simulink model "DR18E_Testpult"  (R2017a)
settings: Solver=ode1  StartTime=0.0  StopTime=Inf  FixedStep=0.001  RelTol=1e-3
PostLoadFcn:
  | , if any(exist('dsrtsu_mdlpostloadfcn', 'file') == [2, 3, 6]), try dsrtsu_mdlpostloadfcn('Execute', bdroot); catch fprintf('Error in PostLoadFcn (dsrtsu_mdlpostloadfcn) for model "%s":\n %s\n', bdroot, lasterr); end, end,
model workspace: external: MATLAB File C:\Users\DeltaRacing\Documents\dSPACE\MABX_DR18E\Model\DR18E_MABX_Parameter.m (data not in the file)
values from neighbouring files (symbols this model uses):
  am = 1/Ts    (= 1)    [DR18E_MABX_Parameter.m]
  bm = K/Ts    (= 0.05)    [DR18E_MABX_Parameter.m]
  cf = 41350    [DR18E_MABX_Parameter.m]
  cr = 41350    [DR18E_MABX_Parameter.m]
  Derating_HV_Battery_Kapa = 1    [DR18E_MABX_Parameter.m]
  Derating_Start_km = 16    [DR18E_MABX_Parameter.m]
  Drive_Mode = 0    [DR18E_MABX_Parameter.m]
  g = 1    [DR18E_MABX_Parameter.m]
  Gas_Modus = 2    [DR18E_MABX_Parameter.m]
  HV_Power_max = 80    [DR18E_MABX_Parameter.m]
  i_Getriebe = 3.3    [DR18E_MABX_Parameter.m]
  i_Lenkgetriebe = 4.32    [DR18E_MABX_Parameter.m]
  K_SET = 1    [DR18E_MABX_Parameter.m]
  Kapazitaet_HV_Battery_kWh = 6.6    [DR18E_MABX_Parameter.m]
  KW_T_Soll = 37    [DR18E_MABX_Parameter.m]
  lf = 1.2    [DR18E_MABX_Parameter.m]
  lr = 1.15    [DR18E_MABX_Parameter.m]
  m = 310    [DR18E_MABX_Parameter.m]
  M_max = 150    [DR18E_MABX_Parameter.m]
  Power_Limit_onoff = 0    [DR18E_MABX_Parameter.m]
  Reifenradius = 0.2351    [DR18E_MABX_Parameter.m]
  Strecke_Endu_km = 22    [DR18E_MABX_Parameter.m]
  TC_Decr_Gas = 0.00005    (= 5e-05)    [DR18E_MABX_Parameter.m]
  TC_Derivative = 0.4    [DR18E_MABX_Parameter.m]
  TC_Incr_Gas = 0.005    [DR18E_MABX_Parameter.m]
  TC_On = 0    [DR18E_MABX_Parameter.m]
  TC_Relay_Off = 0.065    [DR18E_MABX_Parameter.m]
  TC_Relay_On = 0.07    [DR18E_MABX_Parameter.m]
  TV_Mode = 2    [DR18E_MABX_Parameter.m]
  TV_On = 0    [DR18E_MABX_Parameter.m]
  TV_Override = 1    [DR18E_MABX_Parameter.m]
  y = 0.8    [DR18E_MABX_Parameter.m]
undefined symbols (not defined in the file or in its folder): D, DiscIntNeverNeededParam, I, K_OL, P
libraries: simulink x288, rtican x105, rtiusbflightreclib x40, rti1401lib_dio_type3 x10, simulink_extras x10, rti1401lib_adc_type4 x8, rti1401lib_II_base x7
(part 10 of 28)

== system DR18E_Testpult/Verarbeitung/BMS_Monitor ==
  In1 : Inport
  Bus Selector : BusSelector  OutputSignals=BMS,BMS_State,BMS.STK1-5_Temp
  Bus Selector1 : BusSelector  OutputSignals=Cell1-24.Cell1-12.Cell_Voltage_1,Cell1-24.Cell1-12.Cell_Voltage_2,Cell1-24.Cell1-12.Cell_Voltage_3,Cell1-24.Cell1-12.Cell_Voltage_4,Cell1-24.Cell1-12.Cell_Voltage_5,Cell1-24.Cell1-12.Cell_Voltage_6,Cell1-24.Cell1-12.Cell_Voltage_7,Cell1-24.Cell1-12.Cell_Voltage_8,Cell1-24.Cell1-12.Cell_Voltage_9,Cell1-24.Cell1-12.Cell_Voltage_10,Cell1-24.Cell1-12.Cell_Voltage_11,Cell1-24.Cell1-12.Cell_Voltage_12,HV_STR1_MIN_VOLTAGE,HV_STR1_MAX_VOLTAGE
  Bus Selector2 : BusSelector  OutputSignals=HV_Voltage_total,AMS_RelayState,AIR_minus_Status,AIR_plus_Status,Precharge_Relay_Status
  Bus Selector3 : BusSelector  OutputSignals=STK1_Temp1-5.STK1_Temp1,STK1_Temp1-5.STK1_Temp2,STK1_Temp1-5.STK1_Temp3,STK1_Temp1-5.STK1_Temp4,STK1_Temp1-5.STK1_Temp5
  Terminator{,1..23} (24 alike) : Terminator
  wires:
  In1/1 -> Bus Selector/1
  Bus Selector/1 -> Bus Selector1/1  "<BMS>"
  Bus Selector1/1 -> Terminator/1  "<Cell_Voltage_1>"
  Bus Selector1/2 -> Terminator1/1  "<Cell_Voltage_2>"
  Bus Selector1/3 -> Terminator2/1  "<Cell_Voltage_3>"
  Bus Selector1/4 -> Terminator3/1  "<Cell_Voltage_4>"
  Bus Selector1/5 -> Terminator4/1  "<Cell_Voltage_5>"
  Bus Selector1/6 -> Terminator6/1  "<Cell_Voltage_6>"
  Bus Selector1/7 -> Terminator5/1  "<Cell_Voltage_7>"
  Bus Selector1/8 -> Terminator7/1  "<Cell_Voltage_8>"
  Bus Selector1/9 -> Terminator8/1  "<Cell_Voltage_9>"
  Bus Selector1/10 -> Terminator9/1  "<Cell_Voltage_10>"
  Bus Selector1/11 -> Terminator10/1  "<Cell_Voltage_11>"
  Bus Selector1/12 -> Terminator13/1  "<Cell_Voltage_12>"
  Bus Selector1/13 -> Terminator12/1  "<HV_STR1_MIN_VOLTAGE>"
  Bus Selector1/14 -> Terminator11/1  "<HV_STR1_MAX_VOLTAGE>"
  Bus Selector/2 -> Bus Selector2/1  "<BMS_State>"
  Bus Selector2/1 -> Terminator14/1  "<HV_Voltage_total>"
  Bus Selector2/2 -> Terminator15/1  "<AMS_RelayState>"
  Bus Selector2/3 -> Terminator16/1  "<AIR_minus_Status>"
  Bus Selector2/4 -> Terminator17/1  "<AIR_plus_Status>"
  Bus Selector2/5 -> Terminator18/1  "<Precharge_Relay_Status>"
  Bus Selector/3 -> Bus Selector3/1  "<STK1-5_Temp>"
  Bus Selector3/4 -> Terminator22/1  "<STK1_Temp4>"
  Bus Selector3/1 -> Terminator19/1  "<STK1_Temp1>"
  Bus Selector3/2 -> Terminator20/1  "<STK1_Temp2>"
  Bus Selector3/3 -> Terminator21/1  "<STK1_Temp3>"
  Bus Selector3/5 -> Terminator23/1  "<STK1_Temp5>"

== system DR18E_Testpult/Verarbeitung/Bremse ==
  note: Wert: 0...250bar, 0.1 bar Auflösung
  note: 0x00: Alles Ok
      | 0xFF: Error, Sensoren Inplausibel
      | 0xEE: Error, zu hoher Messwert
      | 0xDD: Error, zu niedriger Messwert
      | 0xCC: Error, Kurzschluss
      | 0xBB: Error, Sensor fehlt
  Bremse : Inport
  Gaspedal % : Inport  Port=2
  Bus Selector : BusSelector  OutputSignals=Brake_vorne_1,Brake_rear_2
  Compare To Constant : simulink/Logic and Bit Operations/Compare To Constant  relop=>  const=3  OutDataTypeStr=boolean
  Constant1 : Constant
  FlightRecorder : Subsystem
  FlightRecorder1 : Subsystem
  FlightRecorder2 : Subsystem
  Logical Operator : Logic  Operator=OR  Inputs=1  AllPortsSameDT=off  OutDataTypeStr=boolean
  Mux1 : Mux  Inputs=2
  PT1 Discrete2 : Subsystem
  PlausibilityCheck : Subsystem
  TFilterGas1 : Constant  Value=0.1
  tag scope: Bremse_bin=global, W_Bemse_Inplausibel=global
  wires:
  Mux1/1 -> PT1 Discrete2/1(u)
  Gaspedal %/1 -> PlausibilityCheck/3(Gaspedal %)
  PT1 Discrete2/1(y) -> Compare To Constant/1
  TFilterGas1/1 -> PT1 Discrete2/3(T)
  Constant1/1 -> PT1 Discrete2/2(K)
  Bremse/1 -> Bus Selector/1
  Logical Operator/1 -> FlightRecorder2/1(In1), [Bremse_bin]  "Bremse_bin"
  Compare To Constant/1 -> Logical Operator/1
  Bus Selector/2 -> Mux1/2, PlausibilityCheck/2(Bremsdruck hinten), FlightRecorder1/1(In1)  "<Brake_rear_2>"
  Bus Selector/1 -> PlausibilityCheck/1(Bremsdruck vorne), Mux1/1, FlightRecorder/1(In1)  "<Brake_vorne_1>"
  PlausibilityCheck/1(W_Bremse_Inplausibel) -> [W_Bemse_Inplausibel]

== system DR18E_Testpult/Verarbeitung/DIS ==
  In1 : Inport
  Bus Creator : BusCreator  Inputs=1
  LED Bar Blinken Subsystem : Subsystem
  LED Bar Mode : Constant  OutDataTypeStr=boolean
  LED Bar blinken : Constant  OutDataTypeStr=boolean
  LED Farbe : Constant  Value=3
  Multiport Switch : MultiPortSwitch
  Mux : Mux  Inputs=8
  Out1 : Outport
  wires:
  LED Bar blinken/1 -> LED Bar Blinken Subsystem/1(LED Blinken)
  LED Farbe/1 -> LED Bar Blinken Subsystem/2(LED Farbe)
  LED Bar Blinken Subsystem/1(Out1) -> Mux/1, Mux/2, Mux/3, Mux/4, Mux/5, Mux/6, Mux/8, Mux/7
  Mux/1 -> Multiport Switch/2  "alle LED gleich"
  Bus Creator/1 -> Out1/1
  Multiport Switch/1 -> Bus Creator/1  "LED Bar Vektor"
  LED Bar Mode/1 -> Multiport Switch/1

== system DR18E_Testpult/Verarbeitung/DR18E Torque Control ==
  Gas_0-1 : Inport
  Inputs : Inport  Port=2
  Add : Sum
  Add1 : Sum
  Bus Creator : BusCreator  Inputs=7
  Derating : Subsystem
  FlightRecorder : Subsystem
  Gain2 : Gain  Gain=-g
  Gain4 : Gain  Gain=g
  M Max : Constant  Value=M_max
  M_max : Constant  Value=M_max
  Mux : Mux  Inputs=2
  Power Limit : Subsystem
  Power Limit onoff : Constant  Value=Power_Limit_onoff
  Product : Product
  Product1 : Product
  Saturation : Saturate  UpperLimit=0  LowerLimit=-M_max
  Saturation1 : Saturate  UpperLimit=M_max  LowerLimit=0
  Saturation2 : Saturate  UpperLimit=0  LowerLimit=-M_max
  Saturation3 : Saturate  UpperLimit=M_max  LowerLimit=0
  TC RL : Subsystem
  TC RR : Subsystem
  TC on : Constant  Value=TC_On
  TV RL : Subsystem
  TV RR : Subsystem
  Torque Filter : Subsystem
  MotorTorque Nm : Outport
  M_max/Motor : Outport  Port=2
  Logs2 : Outport  Port=3
  wires:
  Add/1 -> Saturation1/1
  Gain2/1 -> Saturation/1  "Torque_RL-"
  TC RL/2(Motor_Gas_RL) -> Product/2
  Product/1 -> Add/1
  TV RL/1(TV RL Nm) -> Gain2/1
  Saturation/1 -> Add/2
  Gas_0-1/1 -> TC RR/2(Gas_0-1), TC RL/2(Gas_0-1)
  Saturation1/1 -> Power Limit/2(DriverTorqueRequest L [Nm])  "TQ_left_after_TCTV_Nm"
  Saturation3/1 -> Power Limit/3(DriverTorqueRequest R [Nm])  "TQ_right_after_TCTV_Nm"
  Inputs/1 -> Power Limit/4(Inputs), Derating/1(In1), TV RR/1(Inputs), TC RR/3(Inputs), TV RL/1(Inputs), TC RL/3(Inputs)
  Bus Creator/1 -> Logs2/1
  Add1/1 -> Saturation3/1
  TC RR/2(Motor_Gas_RR) -> Product1/2
  Saturation2/1 -> Add1/2
  Product1/1 -> Add1/1
  TC on/1 -> TC RR/1(TC_On), TC RL/1(TC_On)
  TV RR/1(TV RR Nm) -> Gain4/1
  Gain4/1 -> Saturation2/1
  Power Limit/2(LimitedTorque R [Nm]) -> Mux/2
  Power Limit/1(LimitedTorque L [Nm]) -> Mux/1
  Mux/1 -> MotorTorque Nm/1  "Torque_after_PowerLimit_Nm"
  M_max/1 -> Bus Creator/1
  M Max/1 -> FlightRecorder/1(In1), M_max/Motor/1, Product1/1, Product/1  "MmaxproMotor"
  Derating/1(PowerLimit_kW) -> Power Limit/5(Power Limit kW)
  Power Limit onoff/1 -> Power Limit/1(Power Limit onoff)

== system DR18E_Testpult/Verarbeitung/GLV-Undervoltage ==
  GLV-Spannung : Inport
  Bus Selector12 : BusSelector  OutputSignals=RX_GLVAMS.GLV_Voltage_ges
  Cubatt : Constant  Value=0
  Pulse Generator : DiscretePulseGenerator  PulseType=Time based  Period=1  PulseWidth=20
  Switch : Switch  Threshold=11
  GLV-Undervoltage : Outport
  wires:
  Pulse Generator/1 -> Switch/3
  Switch/1 -> GLV-Undervoltage/1  "LV_Undervoltage"
  Cubatt/1 -> Switch/1
  GLV-Spannung/1 -> Bus Selector12/1
  Bus Selector12/1 -> Switch/2  "<GLV_Voltage_ges>"

== system DR18E_Testpult/Verarbeitung/Gaspedal Check ==
  note: 0x00: Alles Ok
      | 0xFF: Error, Sensoren Inplausibel
      | 0xEE: Error, zu hoher Messwert
      | 0xDD: Error, zu niedriger Messwert
      | 0xCC: Error, Kurzschluss
      | 0xBB: Error, Sensor fehlt
      | 0xAA: Sensoren Inplausibel (Erkennung in Software)
  note: 0...100.0% (0.1% Auflösung)
  Gaspedal : Inport
  Add_Software_inplausible_Warning : Subsystem
  Add_Software_inplausible_Warning1 : Subsystem
  Bus Selector : BusSelector  OutputSignals=RX_SensorboardFront.RX_Gas.Throttle_1,RX_SensorboardFront.RX_Gas.Throttle_2,RX_SensorboardFront.RX_Gas.Throttle_1_Status,RX_SensorboardFront.RX_Gas.Throttle_2_Status,RX_SensorboardFront.RX_Gas.RX Timeout Error
  FlightRecorder : Subsystem
  Gas_Modus : Constant  Value=Gas_Modus
  Multiport Switch : MultiPortSwitch  Inputs=2
  PlausibilityCheck : Subsystem
  Saturation 0-1 : Saturate  UpperLimit=1  LowerLimit=0
  Testmodus : Subsystem
  Gas_0-1 : Outport
  tag scope: A_Gas_RX_Timeout=global, W_Gas1_Error=global, W_Gas2_Error=global
  wires:
  Bus Selector/1 -> Testmodus/1(Gas1), PlausibilityCheck/1(Gas1)  "<Throttle_1>"
  Bus Selector/2 -> Testmodus/2(Gas2), PlausibilityCheck/2(Gas2)  "<Throttle_2>"
  Add_Software_inplausible_Warning/1(ErrorCode_Out) -> [W_Gas1_Error]
  Bus Selector/3 -> Add_Software_inplausible_Warning/2(Error_Code)  "<Throttle_1_Status>"
  Add_Software_inplausible_Warning1/1(ErrorCode_Out) -> [W_Gas2_Error]
  Bus Selector/4 -> Add_Software_inplausible_Warning1/2(Error_Code)  "<Throttle_2_Status>"
  Bus Selector/5 -> [A_Gas_RX_Timeout]  "<RX Timeout Error>"
  Gaspedal/1 -> Bus Selector/1
  Saturation 0-1/1 -> Gas_0-1/1, Add_Software_inplausible_Warning1/1(Softw_Plausibel), Add_Software_inplausible_Warning/1(Softw_Plausibel)  "Gas_0-1"
  Multiport Switch/1 -> FlightRecorder/1(In1), Saturation 0-1/1
  Gas_Modus/1 -> Multiport Switch/1
  PlausibilityCheck/1(Gas_0-1_plausibel) -> Multiport Switch/3
  Testmodus/1(Gas_0-1) -> Multiport Switch/2

== system DR18E_Testpult/Verarbeitung/MABX RAM ==
  In1 : Inport
  Add : Sum
  Add1 : Sum
  Add2 : Sum
  Data Type Conversion : DataTypeConversion  OutDataTypeStr=uint16
  Data Type Conversion1 : DataTypeConversion  OutDataTypeStr=uint32
  Data Type Conversion2 : DataTypeConversion  OutDataTypeStr=uint16
  Difference : simulink/Discrete/Difference  ICPrevInput=0.0  OutMin=[]  OutMax=[]  OutDataType=fixdt(1, 16)  OutScaling=2^-10  DoSatur=off
  Difference1 : simulink/Discrete/Difference  ICPrevInput=0.0  OutMin=[]  OutMax=[]  OutDataType=fixdt(1, 16)  OutScaling=2^-10  DoSatur=off
  Difference2 : simulink/Discrete/Difference  ICPrevInput=0.0  OutMin=[]  OutMax=[]  OutDataType=fixdt(1, 16)  OutScaling=2^-10  DoSatur=off
  FlightRecorder5 : Subsystem
  READ Gesamtkilometerzähler Byte 1+2 : rti1401lib_II_base/DS1401_NV_RAM_READ_BL1  DSProperties=struct('RTI',struct('Version',uint32(1),'BlockType',struct('isSLSource',uint8(1),'isSLSink',uint8(0),'isHWSource',uint8(1),'isHWSink',uint8(0),'isSetup',uint8(0),'isInline',uint8(1),'isNonInline',uint8(0),'isInterrupt',uint8(0),'isChannelwise',uint8(0)),'IOBoardType',{{'DS1401','BASE','II'}},'UnitType','NVRAM','Identifier','NVRAMREAD','DialogType','ML','BlockSet','NONE','SlaveProcessor','NONE'))  RTIBlockInterface=struct('OutputPortsWidth',int32(1),'OutputPortsActive',1,'OutputPortsDataType',{{'SS_UINT16'}},'OutputPortsName',{{[' ']}},'BlockDisplay',{{['Read from\nnon-volatile RAM'],'center'}},'IconTransparency','on','InitLevel',3,'SampleTime',{{-1}},'DialogFcn','rti1401baseiinvramreadgui','BlockName',struct('Token',{{'DS1401_NV_RAM_READ_BL1'}}))  RTIBlockParameters=struct('DataType',{{4,'OFF',[1 8]}},'RAMAddress',{{'1','OFF',[0 4095]}},'SampleTime',{{'-1','OFF',[-1 inf]}},'TLCFileName',{{'rti1401base_II_nvram_read','OFF',[]}})  RTISFcnParameters=struct('DataType','int16','RAMAddress','uint32','TLCFileName','char')  RTIBlockParaDefault=struct('DataType',8,'RAMAddress',0,'SampleTime',-1,'TLCFileName','rti1401base_II_nvram_read')
  READ Gesamtkilometerzähler Byte 10+4 : rti1401lib_II_base/DS1401_NV_RAM_READ_BL1  DSProperties=struct('RTI',struct('Version',uint32(1),'BlockType',struct('isSLSource',uint8(1),'isSLSink',uint8(0),'isHWSource',uint8(1),'isHWSink',uint8(0),'isSetup',uint8(0),'isInline',uint8(1),'isNonInline',uint8(0),'isInterrupt',uint8(0),'isChannelwise',uint8(0)),'IOBoardType',{{'DS1401','BASE','II'}},'UnitType','NVRAM','Identifier','NVRAMREAD','DialogType','ML','BlockSet','NONE','SlaveProcessor','NONE'))  RTIBlockInterface=struct('OutputPortsWidth',int32(1),'OutputPortsActive',1,'OutputPortsDataType',{{'SS_UINT32'}},'OutputPortsName',{{[' ']}},'BlockDisplay',{{['Read from\nnon-volatile RAM'],'center'}},'IconTransparency','on','InitLevel',3,'SampleTime',{{-1}},'DialogFcn','rti1401baseiinvramreadgui','BlockName',struct('Token',{{'DS1401_NV_RAM_READ_BL1'}}))  RTIBlockParameters=struct('DataType',{{6,'OFF',[1 8]}},'RAMAddress',{{'10','OFF',[0 4095]}},'SampleTime',{{'-1','OFF',[-1 inf]}},'TLCFileName',{{'rti1401base_II_nvram_read','OFF',[]}})  RTISFcnParameters=struct('DataType','int16','RAMAddress','uint32','TLCFileName','char')  RTIBlockParaDefault=struct('DataType',8,'RAMAddress',0,'SampleTime',-1,'TLCFileName','rti1401base_II_nvram_read')
  READ Tagesenergiezähler Byte 4+2 : rti1401lib_II_base/DS1401_NV_RAM_READ_BL1  DSProperties=struct('RTI',struct('Version',uint32(1),'BlockType',struct('isSLSource',uint8(1),'isSLSink',uint8(0),'isHWSource',uint8(1),'isHWSink',uint8(0),'isSetup',uint8(0),'isInline',uint8(1),'isNonInline',uint8(0),'isInterrupt',uint8(0),'isChannelwise',uint8(0)),'IOBoardType',{{'DS1401','BASE','II'}},'UnitType','NVRAM','Identifier','NVRAMREAD','DialogType','ML','BlockSet','NONE','SlaveProcessor','NONE'))  RTIBlockInterface=struct('OutputPortsWidth',int32(1),'OutputPortsActive',1,'OutputPortsDataType',{{'SS_UINT16'}},'OutputPortsName',{{[' ']}},'BlockDisplay',{{['Read from\nnon-volatile RAM'],'center'}},'IconTransparency','on','InitLevel',3,'SampleTime',{{-1}},'DialogFcn','rti1401baseiinvramreadgui','BlockName',struct('Token',{{'DS1401_NV_RAM_READ_BL1'}}))  RTIBlockParameters=struct('DataType',{{4,'OFF',[1 8]}},'RAMAddress',{{'4','OFF',[0 4095]}},'SampleTime',{{'-1','OFF',[-1 inf]}},'TLCFileName',{{'rti1401base_II_nvram_read','OFF',[]}})  RTISFcnParameters=struct('DataType','int16','RAMAddress','uint32','TLCFileName','char')  RTIBlockParaDefault=struct('DataType',8,'RAMAddress',0,'SampleTime',-1,'TLCFileName','rti1401base_II_nvram_read')
  Reset Tageswerte : Constant  Value=0
  Reset Value : Constant  Value=0  OutDataTypeStr=uint16
  Reset Value1 : Constant  Value=0  OutDataTypeStr=uint16
  Switch : Switch  Criteria=u2 > Threshold
  Switch1 : Switch  Criteria=u2 > Threshold
  WRITE Gesamtmeterzähler m Byte 10+4 : rti1401lib_II_base/DS1401_NV_RAM_WRITE_BL1  DSProperties=struct('RTI',struct('Version',uint32(1),'BlockType',struct('isSLSource',uint8(0),'isSLSink',uint8(1),'isHWSource',uint8(0),'isHWSink',uint8(1),'isSetup',uint8(0),'isInline',uint8(1),'isNonInline',uint8(0),'isInterrupt',uint8(0),'isChannelwise',uint8(0)),'IOBoardType',{{'DS1401','BASE','II'}},'UnitType','NVRAM','Identifier','NVRAMWRITE','DialogType','ML','BlockSet','NONE','SlaveProcessor','NONE'))  RTIBlockInterface=struct('InputPortsWidth',int32(1),'InputPortsActive',1,'InputPortsDataType',{{'SS_UINT32'}},'InputPortsName',{{[' ']}},'BlockDisplay',{{['Write to\nnon-volatile RAM'],'center'}},'IconTransparency','on','InitLevel',3,'SampleTime',{{-1}},'DialogFcn','rti1401baseiinvramwritegui','BlockName',struct('Token',{{'DS1401_NV_RAM_WRITE_BL1'}}))  RTIBlockParameters=struct('DataType',{{6,'OFF',[1 8]}},'RAMAddress',{{'10','OFF',[0 4095]}},'SampleTime',{{'-1','OFF',[-1 inf]}},'TLCFileName',{{'rti1401base_II_nvram_write','OFF',[]}})  RTISFcnParameters=struct('DataType','int16','RAMAddress','uint32','TLCFileName','char')  RTIBlockParaDefault=struct('DataType',8,'RAMAddress',0,'SampleTime',-1,'TLCFileName','rti1401base_II_nvram_write')
  WRITE Tagesmeterzähler Wh Byte 4+2 : rti1401lib_II_base/DS1401_NV_RAM_WRITE_BL1  DSProperties=struct('RTI',struct('Version',uint32(1),'BlockType',struct('isSLSource',uint8(0),'isSLSink',uint8(1),'isHWSource',uint8(0),'isHWSink',uint8(1),'isSetup',uint8(0),'isInline',uint8(1),'isNonInline',uint8(0),'isInterrupt',uint8(0),'isChannelwise',uint8(0)),'IOBoardType',{{'DS1401','BASE','II'}},'UnitType','NVRAM','Identifier','NVRAMWRITE','DialogType','ML','BlockSet','NONE','SlaveProcessor','NONE'))  RTIBlockInterface=struct('InputPortsWidth',int32(1),'InputPortsActive',1,'InputPortsDataType',{{'SS_UINT16'}},'InputPortsName',{{[' ']}},'BlockDisplay',{{['Write to\nnon-volatile RAM'],'center'}},'IconTransparency','on','InitLevel',3,'SampleTime',{{-1}},'DialogFcn','rti1401baseiinvramwritegui','BlockName',struct('Token',{{'DS1401_NV_RAM_WRITE_BL1'}}))  RTIBlockParameters=struct('DataType',{{4,'OFF',[1 8]}},'RAMAddress',{{'4','OFF',[0 4095]}},'SampleTime',{{'-1','OFF',[-1 inf]}},'TLCFileName',{{'rti1401base_II_nvram_write','OFF',[]}})  RTISFcnParameters=struct('DataType','int16','RAMAddress','uint32','TLCFileName','char')  RTIBlockParaDefault=struct('DataType',8,'RAMAddress',0,'SampleTime',-1,'TLCFileName','rti1401base_II_nvram_write')
  WRITE Tagesmeterzähler m Byte 1+2 : rti1401lib_II_base/DS1401_NV_RAM_WRITE_BL1  DSProperties=struct('RTI',struct('Version',uint32(1),'BlockType',struct('isSLSource',uint8(0),'isSLSink',uint8(1),'isHWSource',uint8(0),'isHWSink',uint8(1),'isSetup',uint8(0),'isInline',uint8(1),'isNonInline',uint8(0),'isInterrupt',uint8(0),'isChannelwise',uint8(0)),'IOBoardType',{{'DS1401','BASE','II'}},'UnitType','NVRAM','Identifier','NVRAMWRITE','DialogType','ML','BlockSet','NONE','SlaveProcessor','NONE'))  RTIBlockInterface=struct('InputPortsWidth',int32(1),'InputPortsActive',1,'InputPortsDataType',{{'SS_UINT16'}},'InputPortsName',{{[' ']}},'BlockDisplay',{{['Write to\nnon-volatile RAM'],'center'}},'IconTransparency','on','InitLevel',3,'SampleTime',{{-1}},'DialogFcn','rti1401baseiinvramwritegui','BlockName',struct('Token',{{'DS1401_NV_RAM_WRITE_BL1'}}))  RTIBlockParameters=struct('DataType',{{4,'OFF',[1 8]}},'RAMAddress',{{'1','OFF',[0 4095]}},'SampleTime',{{'-1','OFF',[-1 inf]}},'TLCFileName',{{'rti1401base_II_nvram_write','OFF',[]}})  RTISFcnParameters=struct('DataType','int16','RAMAddress','uint32','TLCFileName','char')  RTIBlockParaDefault=struct('DataType',8,'RAMAddress',0,'SampleTime',-1,'TLCFileName','rti1401base_II_nvram_write')
  TagesmeterMABX_m : Outport
  TagesenergieMABX_Wh : Outport  Port=2
  wires:
  READ Gesamtkilometerzähler Byte 10+4/1 -> Add/2
  Add/1 -> FlightRecorder5/1(In1), WRITE Gesamtmeterzähler m Byte 10+4/1
  [Tagesmeter_s_m] -> Data Type Conversion1/1
  Difference/1 -> Add/1
  Difference1/1 -> Add1/1
  READ Gesamtkilometerzähler Byte 1+2/1 -> Add1/2
  [Tagesmeter_s_m] -> Data Type Conversion/1
  Add1/1 -> Switch/3
  Switch/1 -> TagesmeterMABX_m/1, WRITE Tagesmeterzähler m Byte 1+2/1  "TagesmeterMABX_m"
  Reset Tageswerte/1 -> Switch/2, Switch1/2  "Reset Tageswerte"
  Reset Value/1 -> Switch/1
  Data Type Conversion/1 -> Difference1/1
  Data Type Conversion1/1 -> Difference/1
  READ Tagesenergiezähler Byte 4+2/1 -> Add2/2
  Difference2/1 -> Add2/1
  Switch1/1 -> TagesenergieMABX_Wh/1, WRITE Tagesmeterzähler Wh Byte 4+2/1  "TagesenergieMABX_Wh"
  Add2/1 -> Switch1/3
  Reset Value1/1 -> Switch1/1
  [Tages_HV_energy_con_Wh] -> Data Type Conversion2/1
  Data Type Conversion2/1 -> Difference2/1

== system DR18E_Testpult/Verarbeitung/Precalculations ==
  Drehzahl FL : Inport
  Drehzahl FR : Inport  Port=2
  Drehzahl RL : Inport  Port=3
  Drehzahl RR : Inport  Port=4
  "Inputs Bus " : Inport  Port=5
  Bus Creator : BusCreator  Inputs=3
  FlightRecorder : Subsystem
  FlightRecorder1 : Subsystem
  FlightRecorder2 : Subsystem
  FlightRecorder3 : Subsystem
  FlightRecorder4 : Subsystem
  FlightRecorder5 : Subsystem
  FlightRecorder6 : Subsystem
  Gain : Gain  Gain=1/i_Getriebe
  Gain1 : Gain  Gain=1/i_Getriebe
  Mux : Mux  Inputs=2
  Mux1 : Mux  Inputs=2
  Saturation : Saturate  UpperLimit=1  LowerLimit=0
  Saturation1 : Saturate  UpperLimit=1  LowerLimit=0
  Sum : Sum  Inputs=|++
  Wheelslip Calculation Left : Fcn  Expr=-(u(1) - u(2))/(abs(u(2)) + 0.1)
  Wheelslip Calulation Right : Fcn  Expr=-(u(1) - u(2))/(abs(u(2)) + 0.1)
  größer 0 : Saturate  UpperLimit=100  LowerLimit=0
  kilometer tracking : Subsystem
  "m/s -> km/h" : Gain  Gain=3.6
  rpm-rad/s : Gain  Gain=2*pi/60
  rpm-rad/s1 : Gain  Gain=2*pi/60
  v = omega*r : Gain  Gain=0.5 * 2* pi *(1/60)*Reifenradius
  v_kmh : Outport
  Long_Slip_Left : Outport  Port=2
  Long_Slip_Right : Outport  Port=3
  Outputs Bus : Outport  Port=4
  wires:
  Drehzahl FL/1 -> FlightRecorder4/1(In1), Mux/1, Sum/1  "Drehzahl_FL_rpm"
  Drehzahl FR/1 -> FlightRecorder3/1(In1), Mux1/1, Sum/2  "Drehzahl_FR_rpm"
  Sum/1 -> v = omega*r/1
  v = omega*r/1 -> größer 0/1, "m/s -> km/h"/1
  Mux/1 -> Wheelslip Calculation Left/1
  Drehzahl RL/1 -> rpm-rad/s/1, Gain/1  "Drehzahl_RL_rpm"
  Wheelslip Calculation Left/1 -> Saturation/1
  Mux1/1 -> Wheelslip Calulation Right/1
  Wheelslip Calulation Right/1 -> Saturation1/1
  Drehzahl RR/1 -> rpm-rad/s1/1, Gain1/1  "Drehzahl_RR_rpm"
  Gain/1 -> Mux/2, FlightRecorder1/1(In1)
  Gain1/1 -> Mux1/2, FlightRecorder2/1(In1)
  Saturation/1 -> FlightRecorder5/1(In1), Long_Slip_Left/1
  Saturation1/1 -> Long_Slip_Right/1, FlightRecorder6/1(In1)
  "m/s -> km/h"/1 -> FlightRecorder/1(In1), v_kmh/1
  Bus Creator/1 -> Outputs Bus/1
  "Inputs Bus "/1 -> Bus Creator/3
  rpm-rad/s/1 -> Bus Creator/1  "Drehzahl_RL_rad/s"
  rpm-rad/s1/1 -> Bus Creator/2  "Drehzahl_RR_rad/s"
  größer 0/1 -> kilometer tracking/1(v_ms)

== system DR18E_Testpult/Verarbeitung/SafetyShutdown ==
  TorqueRequestLR : Inport
  Constant : Constant  Value=[0;0]
  Constant1 : Constant  Value=0
  Gas_Modus : Constant  Value=Gas_Modus
  Multiport Switch : MultiPortSwitch  Inputs=2
  Switch : Switch  Criteria=u2 > Threshold
  TorqueRequestLROut : Outport
  wires:
  TorqueRequestLR/1 -> Switch/3
  Constant/1 -> Switch/1
  Switch/1 -> TorqueRequestLROut/1
  Gas_Modus/1 -> Multiport Switch/1
  Constant1/1 -> Multiport Switch/2
  Multiport Switch/1 -> Switch/2
  [Warnings] -> Multiport Switch/3

== system DR18E_Testpult/Verarbeitung/Strom//SOC ==
  HV_Voltage : Inport
  HV_Current : Inport  Port=2
  Discrete-Time Integrator : DiscreteIntegrator  ICPrevOutput=DiscIntNeverNeededParam  ICPrevScaledInput=DiscIntNeverNeededParam
  Discrete-Time Integrator1 : DiscreteIntegrator  ICPrevOutput=DiscIntNeverNeededParam  ICPrevScaledInput=DiscIntNeverNeededParam
  HVIRecorder : Subsystem
  HVURecorder : Subsystem
  Product : Product
  Ws->Wh : Gain  Gain=1/3600
  currentConsumptionRecorder : Subsystem
  powerConsumtionRecorder : Subsystem
  powerRecorder : Subsystem
  HV_Power_Watt : Outport
  tag scope: Tages_HV_energy_con_Wh=global
  wires:
  HV_Voltage/1 -> Product/1, HVURecorder/1(In1)  "HV_Voltage"
  HV_Current/1 -> Discrete-Time Integrator/1, Product/2, HVIRecorder/1(In1)  "HV_Current"
  Discrete-Time Integrator/1 -> currentConsumptionRecorder/1(In1)  "CurrentConsumption"
  Product/1 -> Discrete-Time Integrator1/1, HV_Power_Watt/1, powerRecorder/1(In1)  "HV_Power_Watt"
  Discrete-Time Integrator1/1 -> Ws->Wh/1, powerConsumtionRecorder/1(In1)  "HV_energy_con_Ws"
  Ws->Wh/1 -> [Tages_HV_energy_con_Wh]

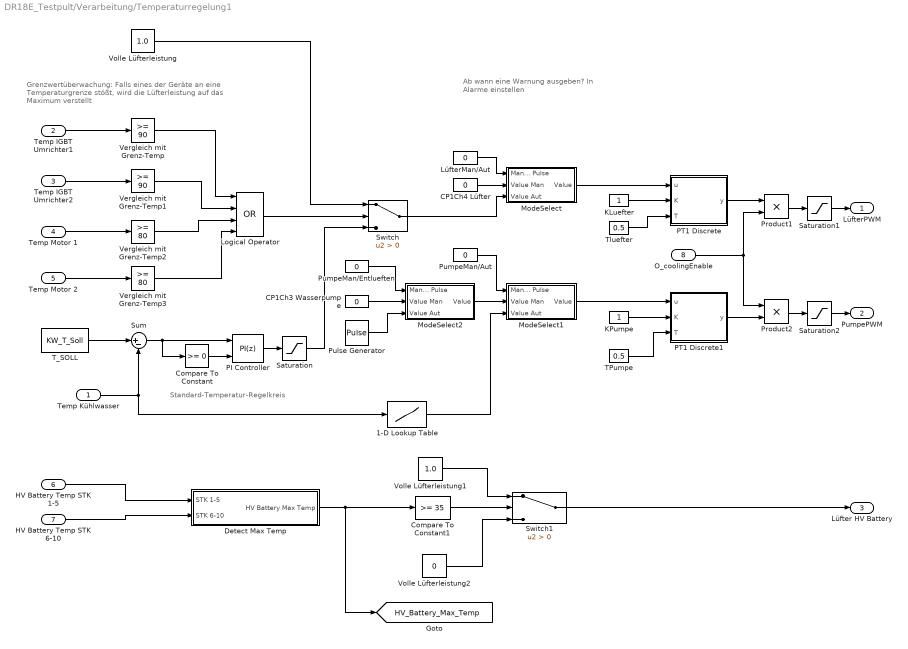
== system DR18E_Testpult/Verarbeitung/Temperaturregelung1 ==
  note: Ab wann eine Warnung ausgeben?
      |
      | In Alarme einstellen
  note: Grenzwertüberwachung:
      | Falls eines der Geräte an eine Temperaturgrenze stößt,
      | wird die Lüfterleistung auf das Maximum verstellt
  note: Standard-Temperatur-Regelkreis
  Temp Kühlwasser : Inport
  Temp IGBT Umrichter1 : Inport  Port=2
  Temp IGBT Umrichter2 : Inport  Port=3
  Temp Motor 1 : Inport  Port=4
  Temp Motor 2 : Inport  Port=5
  HV Battery Temp STK 1-5 : Inport  Port=6
  HV Battery Temp STK 6-10 : Inport  Port=7
  O_coolingEnable : Inport  Port=8
  1-D Lookup Table : Lookup_n-D  NumberOfTableDimensions=1  BreakpointsForDimension1=[0,20,28,35,40,45,50,100]  Table=[0.2,0.2,0.2,0.4,0.6,0.8,1,1]  RndMeth=Simplest  InputSameDT=on
  CP1Ch3 Wasserpumpe : Constant  Value=0
  CP1Ch4 Lüfter : Constant  Value=0
  Compare To Constant : simulink/Logic and Bit Operations/Compare To Constant  relop=>=  const=0  OutDataTypeStr=boolean
  Compare To Constant1 : simulink/Logic and Bit Operations/Compare To Constant  relop=>=  const=35  OutDataTypeStr=boolean
  Detect Max Temp : Subsystem
  KLuefter : Constant
  KPumpe : Constant
  Logical Operator : Logic  Operator=OR  Inputs=4  AllPortsSameDT=off  OutDataTypeStr=boolean
  LüfterMan/Aut : Constant  Value=0
  ModeSelect : Subsystem
  ModeSelect1 : Subsystem
  ModeSelect2 : Subsystem
  PI Controller : simulink/Continuous/PID Controller  Controller=PI  TimeDomain=Discrete-time  SampleTime=0.2  IntegratorMethod=Forward Euler  FilterMethod=Forward Euler  Form=Parallel  UseFilter=on  ControllerParametersSource=internal  P=-0.02  I=-0.01  D=0  N=100  InitialConditionSource=internal  InitialConditionForIntegrator=0  InitialConditionForFilter=0  ExternalReset=level  LimitOutput=off  UpperSaturationLimit=inf  LowerSaturationLimit=-inf  LinearizeAsGain=on  AntiWindupMode=none  Kb=1  TrackingMode=off  Kt=1  PParamMin=[]  PParamMax=[]  IParamMin=[]  IParamMax=[]  DParamMin=[]  DParamMax=[]  NParamMin=[]  NParamMax=[]  KbParamMin=[]  KbParamMax=[]  KtParamMin=[]  KtParamMax=[]  POutMin=[]  POutMax=[]  IOutMin=[]  IOutMax=[]  DOutMin=[]  DOutMax=[]  NOutMin=[]  NOutMax=[]  KbOutMin=[]  KbOutMax=[]  KtOutMin=[]  KtOutMax=[]  IntegratorOutMin=[]  IntegratorOutMax=[]  FilterOutMin=[]  FilterOutMax=[]  SumOutMin=[]  SumOutMax=[]  SumI1OutMin=[]  SumI1OutMax=[]  SumI2OutMin=[]  SumI2OutMax=[]  SumI3OutMin=[]  SumI3OutMax=[]  SumDOutMin=[]  SumDOutMax=[]  SaturationOutMin=[]  SaturationOutMax=[]  IntegratorContinuousStateAttributes=''  IntegratorStateMustResolveToSignalObject=off  IntegratorRTWStateStorageClass=Auto  FilterContinuousStateAttributes=''  FilterStateMustResolveToSignalObject=off  FilterRTWStateStorageClass=Auto  DifferentiatorICPrevScaledInput=0  DifferentiatorOutMin=[]  DifferentiatorOutMax=[]  InitialConditionSetting=State (most efficient)
  PT1 Discrete : Subsystem
  PT1 Discrete1 : Subsystem
  Product1 : Product
  Product2 : Product
  Pulse Generator : DiscretePulseGenerator  PulseType=Time based  Period=3  PulseWidth=50
  PumpeMan/Aut : Constant  Value=0
  PumpeMan/Entlueften : Constant  Value=0
  Saturation : Saturate  UpperLimit=1  LowerLimit=0  LinearizeAsGain=off
  Saturation1 : Saturate  UpperLimit=1  LowerLimit=0
  Saturation2 : Saturate  UpperLimit=1  LowerLimit=0
  Sum : Sum  Inputs=|+-
  Switch : Switch  Criteria=u2 > Threshold
  Switch1 : Switch  Criteria=u2 > Threshold
  TPumpe : Constant  Value=0.5
  T_SOLL : Constant  Value=KW_T_Soll
  Tluefter : Constant  Value=0.5
  Vergleich mit Grenz-Temp : simulink/Logic and Bit Operations/Compare To Constant  relop=>=  const=90  OutDataTypeStr=boolean
  Vergleich mit Grenz-Temp1 : simulink/Logic and Bit Operations/Compare To Constant  relop=>=  const=90  OutDataTypeStr=boolean
  Vergleich mit Grenz-Temp2 : simulink/Logic and Bit Operations/Compare To Constant  relop=>=  const=80  OutDataTypeStr=boolean
  Vergleich mit Grenz-Temp3 : simulink/Logic and Bit Operations/Compare To Constant  relop=>=  const=80  OutDataTypeStr=boolean
  Volle Lüfterleistung : Constant  Value=1.0
  Volle Lüfterleistung1 : Constant  Value=1.0
  Volle Lüfterleistung2 : Constant  Value=0
  LüfterPWM : Outport
  PumpePWM : Outport  Port=2
  Lüfter HV Battery : Outport  Port=3
  tag scope: HV_Battery_Max_Temp=global
  wires:
  T_SOLL/1 -> Sum/1
  Sum/1 -> Compare To Constant/1, PI Controller/1
  PI Controller/1 -> Saturation/1
  Saturation/1 -> Switch/3
  Temp IGBT Umrichter1/1 -> Vergleich mit Grenz-Temp/1
  Temp IGBT Umrichter2/1 -> Vergleich mit Grenz-Temp1/1
  Temp Motor 1/1 -> Vergleich mit Grenz-Temp2/1
  Temp Motor 2/1 -> Vergleich mit Grenz-Temp3/1
  Vergleich mit Grenz-Temp/1 -> Logical Operator/1
  Vergleich mit Grenz-Temp1/1 -> Logical Operator/2
  Vergleich mit Grenz-Temp2/1 -> Logical Operator/3
  Vergleich mit Grenz-Temp3/1 -> Logical Operator/4
  Logical Operator/1 -> Switch/2
  Volle Lüfterleistung/1 -> Switch/1
  Temp Kühlwasser/1 -> 1-D Lookup Table/1, Sum/2
  Compare To Constant/1 -> PI Controller/2
  KLuefter/1 -> PT1 Discrete/2(K)
  Tluefter/1 -> PT1 Discrete/3(T)
  TPumpe/1 -> PT1 Discrete1/3(T)
  KPumpe/1 -> PT1 Discrete1/2(K)
  CP1Ch4 Lüfter/1 -> ModeSelect/2(Value Man)
  LüfterMan/Aut/1 -> ModeSelect/1(Man/Aut Pulse)
  Switch/1 -> ModeSelect/3(Value Aut)
  PumpeMan/Aut/1 -> ModeSelect1/1(Man/Aut Pulse)
  PumpeMan/Entlueften/1 -> ModeSelect2/1(Man/Aut Pulse)
  CP1Ch3 Wasserpumpe/1 -> ModeSelect2/2(Value Man)
  Pulse Generator/1 -> ModeSelect2/3(Value Aut)
  ModeSelect2/1(Value) -> ModeSelect1/2(Value Man)
  ModeSelect/1(Value) -> PT1 Discrete/1(u)
  ModeSelect1/1(Value) -> PT1 Discrete1/1(u)
  O_coolingEnable/1 -> Product2/1, Product1/2
  1-D Lookup Table/1 -> ModeSelect1/3(Value Aut)
  PT1 Discrete/1(y) -> Product1/1
  Product1/1 -> Saturation1/1
  PT1 Discrete1/1(y) -> Product2/2
  Product2/1 -> Saturation2/1
  Saturation1/1 -> LüfterPWM/1
  Saturation2/1 -> PumpePWM/1
  HV Battery Temp STK 1-5/1 -> Detect Max Temp/1(STK 1-5)
  HV Battery Temp STK 6-10/1 -> Detect Max Temp/2(STK 6-10)
  Switch1/1 -> Lüfter HV Battery/1
  Detect Max Temp/1(HV Battery Max Temp) -> [HV_Battery_Max_Temp], Compare To Constant1/1
  Compare To Constant1/1 -> Switch1/2
  Volle Lüfterleistung1/1 -> Switch1/1
  Volle Lüfterleistung2/1 -> Switch1/3

== system DR18E_Testpult/Verarbeitung/Umrichter Init Config ==
  note: Konfiguration des Automatischen Sendeintervalls
  Umrichter 1 Init Config : Subsystem
  Umrichter 2 Init Config : Subsystem

== system DR18E_Testpult/Verarbeitung/Vehicle State Machine ==
  In1 : Inport
  Bus Creator : BusCreator  Inputs=20
  Bus Creator1 : BusCreator  Inputs=4
  Bus Creator2 : BusCreator  Inputs=2
  Bus Creator3 : BusCreator  Inputs=2
  Bus Creator4 : BusCreator  Inputs=2
  Bus Selector1 : BusSelector  OutputSignals=RX_SensorboardMitte.Starttaster
  Bus Selector2 : BusSelector  OutputSignals=A_BSPD,A_BRAKE_OVERTRAVEL,A_NOT_COCKPIT,A_NOT_LINKS,A_NOT_RECHTS,A_AMS_out,A_IMD_out,A_HVD
  Bus Selector3 : BusSelector  OutputSignals=Umrichter.U1.UDC_V,BMS_State.HV_Voltage_total,MicroAutoBox.DI.P2Ch7_IMDAMS_Reset
  Bus Selector4 : BusSelector  OutputSignals=BMS_State.AIR_minus_Status,BMS_State.AIR_plus_Status
  Detect Rise Positive : simulink/Logic and Bit Operations/Detect Rise Positive  vinit=0  InputProcessing=Inherited  OutDataTypeStr=boolean
  Drive_Mode : Constant  Value=Drive_Mode
  Fahrzeugsteuerung : Stateflow chart  TreatAsAtomicUnit=on
  FlightRecorder : Subsystem
  FlightRecorder1 : Subsystem
  Logical Operator4 : Logic  Operator=NOT  AllPortsSameDT=off  OutDataTypeStr=boolean
  Outputs : Outport
  wires:
  Bus Selector3/3 -> Logical Operator4/1  "<P2Ch7_IMDAMS_Reset>"
  Bus Selector3/2 -> Fahrzeugsteuerung/19(I_U_Batt)  "<HV_Voltage_total>"
  Bus Selector2/2 -> Fahrzeugsteuerung/11(A_BRAKE_OVERTRAVEL)  "<A_BRAKE_OVERTRAVEL>"
  Bus Selector1/1 -> Detect Rise Positive/1  "<Starttaster>"
  [U1config_TXZeiten] -> Fahrzeugsteuerung/6(I_vecU1config_TXZeiten)
  [U2config_TXZeiten] -> Fahrzeugsteuerung/8(I_vecU2config_TXZeiten)
  [U1config_TXRegister] -> Fahrzeugsteuerung/5(I_vecU1config_TXRegister)
  Detect Rise Positive/1 -> Fahrzeugsteuerung/1(I_StartButton)
  [U2config_TXRegister] -> Fahrzeugsteuerung/7(I_vecU2config_TXRegister)
  In1/1 -> Bus Selector3/1, Bus Selector4/1, Bus Selector1/1
  Bus Creator/1 -> Outputs/1  "Outputs_StateMachine"
  Fahrzeugsteuerung/13(O_InverterFRE) -> Bus Creator/8
  Fahrzeugsteuerung/15(O_InvertersTXActive) -> Bus Creator/10
  Fahrzeugsteuerung/17(O_U1Init_Reg) -> Bus Creator1/1
  Fahrzeugsteuerung/18(O_U1Init_Zeit) -> Bus Creator1/2
  Fahrzeugsteuerung/19(O_U2Init_Reg) -> Bus Creator1/3
  Fahrzeugsteuerung/20(O_U2Init_Zeit) -> Bus Creator1/4
  Bus Creator1/1 -> Bus Creator/11  "UmrichterInit"
  Bus Creator2/1 -> Bus Creator/1  "UniversalTX"
  Fahrzeugsteuerung/6(O_Sicherheitskreis_Enable) -> Bus Creator/2
  Fahrzeugsteuerung/7(O_Precharge_Enable) -> Bus Creator/3
  Fahrzeugsteuerung/8(O_ErrorNr) -> FlightRecorder1/1(In1), Bus Creator/4
  Fahrzeugsteuerung/9(O_fBlink_Start) -> Bus Creator/5
  Fahrzeugsteuerung/10(O_State) -> FlightRecorder/1(In1), Bus Creator/6
  Fahrzeugsteuerung/2(O_U1_RegID) -> Bus Creator3/1
  Fahrzeugsteuerung/3(O_U2_RegID) -> Bus Creator3/2
  Bus Creator3/1 -> Bus Creator2/1  "RegID_L_R"
  Fahrzeugsteuerung/4(O_U2_Value32) -> Bus Creator4/1
  Fahrzeugsteuerung/5(O_U1_Value32) -> Bus Creator4/2
  Bus Creator4/1 -> Bus Creator2/2  "Value32_L_R"
  Fahrzeugsteuerung/21(O_Inverter_TX_Mode) -> Bus Creator/13
  Bus Selector3/1 -> Fahrzeugsteuerung/18(I_U_Zwischenkreis)  "<UDC_V>"
  Fahrzeugsteuerung/22(O_SoundEnable) -> Bus Creator/14
  Fahrzeugsteuerung/23(O_SoundPlayChannel) -> Bus Creator/15
  Fahrzeugsteuerung/24(O_SpeakerEnable) -> Bus Creator/16
  Bus Selector4/1 -> Fahrzeugsteuerung/3(AIR_L)  "<AIR_minus_Status>"
  Bus Selector4/2 -> Fahrzeugsteuerung/4(AIR_R)  "<AIR_plus_Status>"
  [Sicherheitskreis] -> Fahrzeugsteuerung/2(I_Sicherheitskreis)  "I_Sicherheitskreis_in"
  [vec_Sicherheitskreis] -> Bus Selector2/1
  Bus Selector2/3 -> Fahrzeugsteuerung/12(A_NOT_COCKPIT)  "<A_NOT_COCKPIT>"
  Bus Selector2/4 -> Fahrzeugsteuerung/13(A_NOT_LINKS)  "<A_NOT_LINKS>"
  Bus Selector2/5 -> Fahrzeugsteuerung/14(A_NOT_RECHTS)  "<A_NOT_RECHTS>"
  Bus Selector2/6 -> Fahrzeugsteuerung/15(A_AMS)  "<A_AMS_out>"
  Bus Selector2/7 -> Fahrzeugsteuerung/16(A_IMD)  "<A_IMD_out>"
  Bus Selector2/8 -> Fahrzeugsteuerung/17(A_HVD)  "<A_HVD>"
  Bus Selector2/1 -> Fahrzeugsteuerung/10(A_BPD)  "<A_BSPD>"
  Logical Operator4/1 -> Fahrzeugsteuerung/20(I_AMS_IMD_Reset)
  Fahrzeugsteuerung/25(O_coolingEnable) -> Bus Creator/19
  Drive_Mode/1 -> Fahrzeugsteuerung/21(I_Drive_Mode)
  [Bremse_bin] -> Fahrzeugsteuerung/22(I_Bremse_bin)

== system DR18E_Testpult/Ausgabe/AMS/Transmit OK Detection3 ==
  note: This subsystem surveys if the sending of the TX message is successful and if it meets the
      | requirements concerning the regularity of the sending.
      |
      | If for 5 consecutive execution steps the message could not be successfully sent the 'TX Warn'
      | output is set to 1. Also, the message is expected to be sent every 50 ms approximatively. If this
      | condition is not met 5 times consecutively the 'TX Warn' output is set to 1.
  TX status : Inport
  TX delta time : Inport  Port=2
  Delta time limit : Constant  Value=0.055
  Delta time limit exceeded : RelationalOperator  RndMeth=Nearest  InputSameDT=on
  Mem{1..4} (4 alike) : Memory
  OR : Logic  Operator=OR
  Prev. msg. not sent : RelationalOperator  Operator=~=  RndMeth=Nearest  InputSameDT=on
  Prev. msg. sent value : Constant
  Warn : Logic  Inputs=5
  TX Warn : Outport
  wires:
  TX delta time/1 -> Delta time limit exceeded/1
  Delta time limit/1 -> Delta time limit exceeded/2
  Prev. msg. sent value/1 -> Prev. msg. not sent/2
  TX status/1 -> Prev. msg. not sent/1
  Prev. msg. not sent/1 -> OR/1
  Delta time limit exceeded/1 -> OR/2
  OR/1 -> Mem1/1, Warn/1
  Mem1/1 -> Mem2/1, Warn/2
  Mem2/1 -> Mem3/1, Warn/3
  Mem3/1 -> Mem4/1, Warn/4
  Mem4/1 -> Warn/5
  Warn/1 -> TX Warn/1

== system DR18E_Testpult/Ausgabe/CANIO/Transmit OK Detection ==
  note: This subsystem surveys if the sending of the TX message is successful and if it meets the
      | requirements concerning the regularity of the sending.
      |
      | If for 5 consecutive execution steps the message could not be successfully sent the 'TX Warn'
      | output is set to 1. Also, the message is expected to be sent every 50 ms approximatively. If this
      | condition is not met 5 times consecutively the 'TX Warn' output is set to 1.
  TX status : Inport
  TX delta time : Inport  Port=2
  Delta time limit : Constant  Value=0.055
  Delta time limit exceeded : RelationalOperator  RndMeth=Nearest  InputSameDT=on
  Mem{1..4} (4 alike) : Memory
  OR : Logic  Operator=OR
  Prev. msg. not sent : RelationalOperator  Operator=~=  RndMeth=Nearest  InputSameDT=on
  Prev. msg. sent value : Constant
  Warn : Logic  Inputs=5
  TX Warn : Outport
  wires:
  TX delta time/1 -> Delta time limit exceeded/1
  Delta time limit/1 -> Delta time limit exceeded/2
  Prev. msg. sent value/1 -> Prev. msg. not sent/2
  TX status/1 -> Prev. msg. not sent/1
  Prev. msg. not sent/1 -> OR/1
  Delta time limit exceeded/1 -> OR/2
  OR/1 -> Mem1/1, Warn/1
  Mem1/1 -> Mem2/1, Warn/2
  Mem2/1 -> Mem3/1, Warn/3
  Mem3/1 -> Mem4/1, Warn/4
  Mem4/1 -> Warn/5
  Warn/1 -> TX Warn/1

== system DR18E_Testpult/Ausgabe/CANIO/Transmit OK Detection1 ==
  note: This subsystem surveys if the sending of the TX message is successful and if it meets the
      | requirements concerning the regularity of the sending.
      |
      | If for 5 consecutive execution steps the message could not be successfully sent the 'TX Warn'
      | output is set to 1. Also, the message is expected to be sent every 50 ms approximatively. If this
      | condition is not met 5 times consecutively the 'TX Warn' output is set to 1.
  TX status : Inport
  TX delta time : Inport  Port=2
  Delta time limit : Constant  Value=0.055
  Delta time limit exceeded : RelationalOperator  RndMeth=Nearest  InputSameDT=on
  Mem{1..4} (4 alike) : Memory
  OR : Logic  Operator=OR
  Prev. msg. not sent : RelationalOperator  Operator=~=  RndMeth=Nearest  InputSameDT=on
  Prev. msg. sent value : Constant
  Warn : Logic  Inputs=5
  TX Warn : Outport
  wires:
  TX delta time/1 -> Delta time limit exceeded/1
  Delta time limit/1 -> Delta time limit exceeded/2
  Prev. msg. sent value/1 -> Prev. msg. not sent/2
  TX status/1 -> Prev. msg. not sent/1
  Prev. msg. not sent/1 -> OR/1
  Delta time limit exceeded/1 -> OR/2
  OR/1 -> Mem1/1, Warn/1
  Mem1/1 -> Mem2/1, Warn/2
  Mem2/1 -> Mem3/1, Warn/3
  Mem3/1 -> Mem4/1, Warn/4
  Mem4/1 -> Warn/5
  Warn/1 -> TX Warn/1

== system DR18E_Testpult/Ausgabe/CANIO/Transmit OK Detection2 ==
  note: This subsystem surveys if the sending of the TX message is successful and if it meets the
      | requirements concerning the regularity of the sending.
      |
      | If for 5 consecutive execution steps the message could not be successfully sent the 'TX Warn'
      | output is set to 1. Also, the message is expected to be sent every 50 ms approximatively. If this
      | condition is not met 5 times consecutively the 'TX Warn' output is set to 1.
  TX status : Inport
  TX delta time : Inport  Port=2
  Delta time limit : Constant  Value=0.055
  Delta time limit exceeded : RelationalOperator  RndMeth=Nearest  InputSameDT=on
  Mem{1..4} (4 alike) : Memory
  OR : Logic  Operator=OR
  Prev. msg. not sent : RelationalOperator  Operator=~=  RndMeth=Nearest  InputSameDT=on
  Prev. msg. sent value : Constant
  Warn : Logic  Inputs=5
  TX Warn : Outport
  wires:
  TX delta time/1 -> Delta time limit exceeded/1
  Delta time limit/1 -> Delta time limit exceeded/2
  Prev. msg. sent value/1 -> Prev. msg. not sent/2
  TX status/1 -> Prev. msg. not sent/1
  Prev. msg. not sent/1 -> OR/1
  Delta time limit exceeded/1 -> OR/2
  OR/1 -> Mem1/1, Warn/1
  Mem1/1 -> Mem2/1, Warn/2
  Mem2/1 -> Mem3/1, Warn/3
  Mem3/1 -> Mem4/1, Warn/4
  Mem4/1 -> Warn/5
  Warn/1 -> TX Warn/1

== system DR18E_Testpult/Ausgabe/CANIO/Transmit OK Detection3 ==
  note: This subsystem surveys if the sending of the TX message is successful and if it meets the
      | requirements concerning the regularity of the sending.
      |
      | If for 5 consecutive execution steps the message could not be successfully sent the 'TX Warn'
      | output is set to 1. Also, the message is expected to be sent every 50 ms approximatively. If this
      | condition is not met 5 times consecutively the 'TX Warn' output is set to 1.
  TX status : Inport
  TX delta time : Inport  Port=2
  Delta time limit : Constant  Value=0.055
  Delta time limit exceeded : RelationalOperator  RndMeth=Nearest  InputSameDT=on
  Mem{1..4} (4 alike) : Memory
  OR : Logic  Operator=OR
  Prev. msg. not sent : RelationalOperator  Operator=~=  RndMeth=Nearest  InputSameDT=on
  Prev. msg. sent value : Constant
  Warn : Logic  Inputs=5
  TX Warn : Outport
  wires:
  TX delta time/1 -> Delta time limit exceeded/1
  Delta time limit/1 -> Delta time limit exceeded/2
  Prev. msg. sent value/1 -> Prev. msg. not sent/2
  TX status/1 -> Prev. msg. not sent/1
  Prev. msg. not sent/1 -> OR/1
  Delta time limit exceeded/1 -> OR/2
  OR/1 -> Mem1/1, Warn/1
  Mem1/1 -> Mem2/1, Warn/2
  Mem2/1 -> Mem3/1, Warn/3
  Mem3/1 -> Mem4/1, Warn/4
  Mem4/1 -> Warn/5
  Warn/1 -> TX Warn/1

== system DR18E_Testpult/Ausgabe/CANIO/Transmit OK Detection4 ==
  note: This subsystem surveys if the sending of the TX message is successful and if it meets the
      | requirements concerning the regularity of the sending.
      |
      | If for 5 consecutive execution steps the message could not be successfully sent the 'TX Warn'
      | output is set to 1. Also, the message is expected to be sent every 50 ms approximatively. If this
      | condition is not met 5 times consecutively the 'TX Warn' output is set to 1.
  TX status : Inport
  TX delta time : Inport  Port=2
  Delta time limit : Constant  Value=0.055
  Delta time limit exceeded : RelationalOperator  RndMeth=Nearest  InputSameDT=on
  Mem{1..4} (4 alike) : Memory
  OR : Logic  Operator=OR
  Prev. msg. not sent : RelationalOperator  Operator=~=  RndMeth=Nearest  InputSameDT=on
  Prev. msg. sent value : Constant
  Warn : Logic  Inputs=5
  TX Warn : Outport
  wires:
  TX delta time/1 -> Delta time limit exceeded/1
  Delta time limit/1 -> Delta time limit exceeded/2
  Prev. msg. sent value/1 -> Prev. msg. not sent/2
  TX status/1 -> Prev. msg. not sent/1
  Prev. msg. not sent/1 -> OR/1
  Delta time limit exceeded/1 -> OR/2
  OR/1 -> Mem1/1, Warn/1
  Mem1/1 -> Mem2/1, Warn/2
  Mem2/1 -> Mem3/1, Warn/3
  Mem3/1 -> Mem4/1, Warn/4
  Mem4/1 -> Warn/5
  Warn/1 -> TX Warn/1

== system DR18E_Testpult/Ausgabe/CANIO/Transmit OK Detection5 ==
  note: This subsystem surveys if the sending of the TX message is successful and if it meets the
      | requirements concerning the regularity of the sending.
      |
      | If for 5 consecutive execution steps the message could not be successfully sent the 'TX Warn'
      | output is set to 1. Also, the message is expected to be sent every 50 ms approximatively. If this
      | condition is not met 5 times consecutively the 'TX Warn' output is set to 1.
  TX status : Inport
  TX delta time : Inport  Port=2
  Delta time limit : Constant  Value=0.055
  Delta time limit exceeded : RelationalOperator  RndMeth=Nearest  InputSameDT=on
  Mem{1..4} (4 alike) : Memory
  OR : Logic  Operator=OR
  Prev. msg. not sent : RelationalOperator  Operator=~=  RndMeth=Nearest  InputSameDT=on
  Prev. msg. sent value : Constant
  Warn : Logic  Inputs=5
  TX Warn : Outport
  wires:
  TX delta time/1 -> Delta time limit exceeded/1
  Delta time limit/1 -> Delta time limit exceeded/2
  Prev. msg. sent value/1 -> Prev. msg. not sent/2
  TX status/1 -> Prev. msg. not sent/1
  Prev. msg. not sent/1 -> OR/1
  Delta time limit exceeded/1 -> OR/2
  OR/1 -> Mem1/1, Warn/1
  Mem1/1 -> Mem2/1, Warn/2
  Mem2/1 -> Mem3/1, Warn/3
  Mem3/1 -> Mem4/1, Warn/4
  Mem4/1 -> Warn/5
  Warn/1 -> TX Warn/1

== system DR18E_Testpult/Ausgabe/CANIO/Transmit OK Detection6 ==
  note: This subsystem surveys if the sending of the TX message is successful and if it meets the
      | requirements concerning the regularity of the sending.
      |
      | If for 5 consecutive execution steps the message could not be successfully sent the 'TX Warn'
      | output is set to 1. Also, the message is expected to be sent every 50 ms approximatively. If this
      | condition is not met 5 times consecutively the 'TX Warn' output is set to 1.
  TX status : Inport
  TX delta time : Inport  Port=2
  Delta time limit : Constant  Value=0.055
  Delta time limit exceeded : RelationalOperator  RndMeth=Nearest  InputSameDT=on
  Mem{1..4} (4 alike) : Memory
  OR : Logic  Operator=OR
  Prev. msg. not sent : RelationalOperator  Operator=~=  RndMeth=Nearest  InputSameDT=on
  Prev. msg. sent value : Constant
  Warn : Logic  Inputs=5
  TX Warn : Outport
  wires:
  TX delta time/1 -> Delta time limit exceeded/1
  Delta time limit/1 -> Delta time limit exceeded/2
  Prev. msg. sent value/1 -> Prev. msg. not sent/2
  TX status/1 -> Prev. msg. not sent/1
  Prev. msg. not sent/1 -> OR/1
  Delta time limit exceeded/1 -> OR/2
  OR/1 -> Mem1/1, Warn/1
  Mem1/1 -> Mem2/1, Warn/2
  Mem2/1 -> Mem3/1, Warn/3
  Mem3/1 -> Mem4/1, Warn/4
  Mem4/1 -> Warn/5
  Warn/1 -> TX Warn/1

== system DR18E_Testpult/Ausgabe/Diagnose/Transmit OK Detection1 ==
  note: This subsystem surveys if the sending of the TX message is successful and if it meets the
      | requirements concerning the regularity of the sending.
      |
      | If for 5 consecutive execution steps the message could not be successfully sent the 'TX Warn'
      | output is set to 1. Also, the message is expected to be sent every 50 ms approximatively. If this
      | condition is not met 5 times consecutively the 'TX Warn' output is set to 1.
  TX status : Inport
  TX delta time : Inport  Port=2
  Delta time limit : Constant  Value=0.055
  Delta time limit exceeded : RelationalOperator  RndMeth=Nearest  InputSameDT=on
  Mem{1..4} (4 alike) : Memory
  OR : Logic  Operator=OR
  Prev. msg. not sent : RelationalOperator  Operator=~=  RndMeth=Nearest  InputSameDT=on
  Prev. msg. sent value : Constant
  Warn : Logic  Inputs=5
  TX Warn : Outport
  wires:
  TX delta time/1 -> Delta time limit exceeded/1
  Delta time limit/1 -> Delta time limit exceeded/2
  Prev. msg. sent value/1 -> Prev. msg. not sent/2
  TX status/1 -> Prev. msg. not sent/1
  Prev. msg. not sent/1 -> OR/1
  Delta time limit exceeded/1 -> OR/2
  OR/1 -> Mem1/1, Warn/1
  Mem1/1 -> Mem2/1, Warn/2
  Mem2/1 -> Mem3/1, Warn/3
  Mem3/1 -> Mem4/1, Warn/4
  Mem4/1 -> Warn/5
  Warn/1 -> TX Warn/1

== system DR18E_Testpult/Ausgabe/Diagnose/Transmit OK Detection2 ==
  note: This subsystem surveys if the sending of the TX message is successful and if it meets the
      | requirements concerning the regularity of the sending.
      |
      | If for 5 consecutive execution steps the message could not be successfully sent the 'TX Warn'
      | output is set to 1. Also, the message is expected to be sent every 50 ms approximatively. If this
      | condition is not met 5 times consecutively the 'TX Warn' output is set to 1.
  TX status : Inport
  TX delta time : Inport  Port=2
  Delta time limit : Constant  Value=0.055
  Delta time limit exceeded : RelationalOperator  RndMeth=Nearest  InputSameDT=on
  Mem{1..4} (4 alike) : Memory
  OR : Logic  Operator=OR
  Prev. msg. not sent : RelationalOperator  Operator=~=  RndMeth=Nearest  InputSameDT=on
  Prev. msg. sent value : Constant
  Warn : Logic  Inputs=5
  TX Warn : Outport
  wires:
  TX delta time/1 -> Delta time limit exceeded/1
  Delta time limit/1 -> Delta time limit exceeded/2
  Prev. msg. sent value/1 -> Prev. msg. not sent/2
  TX status/1 -> Prev. msg. not sent/1
  Prev. msg. not sent/1 -> OR/1
  Delta time limit exceeded/1 -> OR/2
  OR/1 -> Mem1/1, Warn/1
  Mem1/1 -> Mem2/1, Warn/2
  Mem2/1 -> Mem3/1, Warn/3
  Mem3/1 -> Mem4/1, Warn/4
  Mem4/1 -> Warn/5
  Warn/1 -> TX Warn/1
